simulink model "CPGGait2"  (R2021a)
settings: Solver=FixedStepDiscrete  StartTime=0.0  StopTime=30  FixedStep=deltaT  RelTol=1e-3  EnableMultiTasking=on
InitFcn:
  | deltaT = 0.02; % this model runs at 50 Hz
  | 
  | DEVICENAME  = 'COM4'; % COM port that USB2Dynamixel is plugged into
  | % NOTE: go to Device Manager to make sure device name is correct
  | 
  | lib_name = ''; % initialize library name
  | % get library name based on computer:
  | if strcmp(computer, 'PCWIN')
  |   lib_name = 'dxl_x86_c';
  | elseif strcmp(computer, 'PCWIN64')
  |   lib_name = 'dxl_x64_c';
  | elseif strcmp(computer, 'GLNX86')
  |   lib_name = 'libdxl_x86_c';
  | elseif strcmp(computer, 'GLNXA64')
  |   lib_name = 'libdxl_x64_c';
  | elseif strcmp(computer, 'MACI64')
  |   lib_name = 'libdxl_mac_c';
  | end
  | 
  | % Load Libraries
  | if ~libisloaded(lib_name)
  |     [notfound, warnings] = loadlibrary(lib_name, 'dynamixel_sdk.h', 'addheader', 'port_handler.h', 'addheader', 'packet_handler.h', 'addheader','group_sync_write.h');
  | end
  | 
  | % Control table address
  | ADDR_MX_TORQUE_ENABLE       = 24;           % Control table address is different in Dynamixel model
  | ADDR_MX_GOAL_POSITION       = 30;
  | ADDR_MX_PRESENT_POSITION    = 36;
  | 
  | % Data Byte Length
  | LEN_MX_GOAL_POSITION        = 2;
  | 
  | % Protocol version
  | PROTOCOL_VERSION            = 1.0;          % See which protocol version is used in the Dynamixel
  | 
  | % Default setting
  | BAUDRATE                    = 1000000;
  | 
  | TORQUE_ENABLE               = 1;            % Value for enabling the torque
  | TORQUE_DISABLE              = 0;            % Value for disabling the torque
  | DXL_MINIMUM_POSITION_VALUE  = 100;          % Dynamixel will rotate between this value
  | DXL_MAXIMUM_POSITION_VALUE  = 500;         % and this value (note that the Dynamixel would not move when the position value is out of movable range. Check e-manual about the range of the Dynamixel you use.)
  | DXL_MOVING_STATUS_THRESHOLD = 10;           % Dynamixel moving status threshold
  | 
  | COMM_SUCCESS                = 0;            % Communication Success result value
  | COMM_TX_FAIL                = -1001;        % Communication Tx Failed
  | 
  | % Initialize PortHandler Structs
  | % Set the port path
  | % Get methods and members of PortHandlerLinux or PortHandlerWindows
  | port_num = portHandler(DEVICENAME);
  | 
  | % Initialize PacketHandler Structs
  | packetHandler();
  | 
  | dxl_comm_result = COMM_TX_FAIL;             % Communication result
  | 
  | dxl_error = 0;                              % Dynamixel error
  | dxl_present_position = 0;                   % Present position
  | 
  | % Initialize Groupsyncwrite instance
  | group_num = groupSyncWrite(port_num, PROTOCOL_VERSION, ADDR_MX_GOAL_POSITION, LEN_MX_GOAL_POSITION);
  | 
  | % Open port
  | if (openPort(port_num))
  |     fprintf('Succeeded to open the port!\n');
  | else
  |     unloadlibrary(lib_name);
  |     fprintf('Failed to open the port!\n');
  |     input('Press any key to terminate...\n');
  |     dxl_error = 1000;
  |     return;
  | end
  | 
  | % Set port baudrate
  | if (setBaudRate(port_num, BAUDRATE))
  |     fprintf('Succeeded to change the baudrate!\n');
  | else
  |     unloadlibrary(lib_name);
  |     fprintf('Failed to change the baudrate!\n');
  |     input('Press any key to terminate...\n');
  |     dxl_error = 2000;
  |     return;
  | end
  | 
  | % set ID numbers of the the Dynamixels to be controlled:
  | % (even numbers are left side of body, odd numbers are right side)
  | ID01                     = 1;            % Dynamixel IDs for sagittal shoulders
  | ID02                     = 2;
  | ID03                     = 3;            % Dynamixel IDs for frontal shoulders
  | ID04                     = 4;
  | ID05                     = 5;            % Dynamixel IDs for elbows
  | ID06                     = 6;
  | ID07                     = 7;            % Dynamixel IDs for transverse hips
  | ID08                     = 8;
  | ID09                     = 9;            % Dynamixel IDs for frontal hips
  | ID10                     = 10;
  | ID11                     = 11;            % Dynamixel IDs for sagittal hips
  | ID12                     = 12;
  | ID13                     = 13;            % Dynamixel IDs for knees
  | ID14                     = 14;
  | ID15                     = 15;            % Dynamixel IDs for sagittal ankles
  | ID16                     = 16;
  | ID17                     = 17;            % Dynamixel IDs for frontal ankles
  | ID18                     = 18;
  | 
  | %% Enable Dynamixel Torques and connect Dynamixels
  | write1ByteTxRx(port_num, PROTOCOL_VERSION, ID01, ADDR_MX_TORQUE_ENABLE, TORQUE_ENABLE);
  | write1ByteTxRx(port_num, PROTOCOL_VERSION, ID02, ADDR_MX_TORQUE_ENABLE, TORQUE_ENABLE);
  | write1ByteTxRx(port_num, PROTOCOL_VERSION, ID03, ADDR_MX_TORQUE_ENABLE, TORQUE_ENABLE);
  | write1ByteTxRx(port_num, PROTOCOL_VERSION, ID04, ADDR_MX_TORQUE_ENABLE, TORQUE_ENABLE);
  | write1ByteTxRx(port_num, PROTOCOL_VERSION, ID05, ADDR_MX_TORQUE_ENABLE, TORQUE_ENABLE);
  | write1ByteTxRx(port_num, PROTOCOL_VERSION, ID06, ADDR_MX_TORQUE_ENABLE, TORQUE_ENABLE);
  | write1ByteTxRx(port_num, PROTOCOL_VERSION, ID07, ADDR_MX_TORQUE_ENABLE, TORQUE_ENABLE);
  | write1ByteTxRx(port_num, PROTOCOL_VERSION, ID08, ADDR_MX_TORQUE_ENABLE, TORQUE_ENABLE);
  | write1ByteTxRx(port_num, PROTOCOL_VERSION, ID09, ADDR_MX_TORQUE_ENABLE, TORQUE_ENABLE);
  | write1ByteTxRx(port_num, PROTOCOL_VERSION, ID10, ADDR_MX_TORQUE_ENABLE, TORQUE_ENABLE);
  | write1ByteTxRx(port_num, PROTOCOL_VERSION, ID11, ADDR_MX_TORQUE_ENABLE, TORQUE_ENABLE);
  | write1ByteTxRx(port_num, PROTOCOL_VERSION, ID12, ADDR_MX_TORQUE_ENABLE, TORQUE_ENABLE);
  | write1ByteTxRx(port_num, PROTOCOL_VERSION, ID13, ADDR_MX_TORQUE_ENABLE, TORQUE_ENABLE);
  | write1ByteTxRx(port_num, PROTOCOL_VERSION, ID14, ADDR_MX_TORQUE_ENABLE, TORQUE_ENABLE);
  | write1ByteTxRx(port_num, PROTOCOL_VERSION, ID15, ADDR_MX_TORQUE_ENABLE, TORQUE_ENABLE);
  | write1ByteTxRx(port_num, PROTOCOL_VERSION, ID16, ADDR_MX_TORQUE_ENABLE, TORQUE_ENABLE);
  | write1ByteTxRx(port_num, PROTOCOL_VERSION, ID17, ADDR_MX_TORQUE_ENABLE, TORQUE_ENABLE);
  | write1ByteTxRx(port_num, PROTOCOL_VERSION, ID18, ADDR_MX_TORQUE_ENABLE, TORQUE_ENABLE);
  | dxl_comm_result = getLastTxRxResult(port_num, PROTOCOL_VERSION);
  | dxl_error = getLastRxPacketError(port_num, PROTOCOL_VERSION);
  | if dxl_comm_result ~= COMM_SUCCESS
  |     fprintf('%s\n', getTxRxResult(PROTOCOL_VERSION, dxl_comm_result));
  | elseif dxl_error ~= 0
  |     fprintf('%s\n', getRxPacketError(PROTOCOL_VERSION, dxl_error));
  | else
  |     fprintf('Dynamixel has been successfully connected \n');
  | end
  | 
  | % the variable 'qinitial' is an 18x1 vector of initial joint angles for the
  | % robot (in DEGREES!); adjust for your robot!
  | if exist('qinitial','var') ~= 1
  | qinitial = (180/pi)*[0.2;1.19321189006954;-1.72642378013908;0.413211890069541;0.15;0;0;-0.15;0.413211890069541;-1.72642378013908;1.19321189006954;0.20;0.1683;0.349;-0.051;0.1683;-0.349;0.997];
  | end
StopFcn:
  | %% Disable Dynamixel Torque and close program
  | write1ByteTxRx(port_num, PROTOCOL_VERSION, ID01, ADDR_MX_TORQUE_ENABLE, TORQUE_DISABLE);
  | write1ByteTxRx(port_num, PROTOCOL_VERSION, ID02, ADDR_MX_TORQUE_ENABLE, TORQUE_DISABLE);
  | write1ByteTxRx(port_num, PROTOCOL_VERSION, ID03, ADDR_MX_TORQUE_ENABLE, TORQUE_DISABLE);
  | write1ByteTxRx(port_num, PROTOCOL_VERSION, ID04, ADDR_MX_TORQUE_ENABLE, TORQUE_DISABLE);
  | write1ByteTxRx(port_num, PROTOCOL_VERSION, ID05, ADDR_MX_TORQUE_ENABLE, TORQUE_DISABLE);
  | write1ByteTxRx(port_num, PROTOCOL_VERSION, ID06, ADDR_MX_TORQUE_ENABLE, TORQUE_DISABLE);
  | write1ByteTxRx(port_num, PROTOCOL_VERSION, ID07, ADDR_MX_TORQUE_ENABLE, TORQUE_DISABLE);
  | write1ByteTxRx(port_num, PROTOCOL_VERSION, ID08, ADDR_MX_TORQUE_ENABLE, TORQUE_DISABLE);
  | write1ByteTxRx(port_num, PROTOCOL_VERSION, ID09, ADDR_MX_TORQUE_ENABLE, TORQUE_DISABLE);
  | write1ByteTxRx(port_num, PROTOCOL_VERSION, ID10, ADDR_MX_TORQUE_ENABLE, TORQUE_DISABLE);
  | write1ByteTxRx(port_num, PROTOCOL_VERSION, ID11, ADDR_MX_TORQUE_ENABLE, TORQUE_DISABLE);
  | write1ByteTxRx(port_num, PROTOCOL_VERSION, ID12, ADDR_MX_TORQUE_ENABLE, TORQUE_DISABLE);
  | write1ByteTxRx(port_num, PROTOCOL_VERSION, ID13, ADDR_MX_TORQUE_ENABLE, TORQUE_DISABLE);
  | write1ByteTxRx(port_num, PROTOCOL_VERSION, ID14, ADDR_MX_TORQUE_ENABLE, TORQUE_DISABLE);
  | write1ByteTxRx(port_num, PROTOCOL_VERSION, ID15, ADDR_MX_TORQUE_ENABLE, TORQUE_DISABLE);
  | write1ByteTxRx(port_num, PROTOCOL_VERSION, ID16, ADDR_MX_TORQUE_ENABLE, TORQUE_DISABLE);
  | write1ByteTxRx(port_num, PROTOCOL_VERSION, ID17, ADDR_MX_TORQUE_ENABLE, TORQUE_DISABLE);
  | write1ByteTxRx(port_num, PROTOCOL_VERSION, ID18, ADDR_MX_TORQUE_ENABLE, TORQUE_DISABLE);
  | dxl_comm_result = getLastTxRxResult(port_num, PROTOCOL_VERSION);
  | dxl_error = getLastRxPacketError(port_num, PROTOCOL_VERSION);
  |    if dxl_comm_result ~= COMM_SUCCESS
  |        fprintf('%s\n', getTxRxResult(PROTOCOL_VERSION, dxl_comm_result));
  |    elseif dxl_error ~= 0
  |        fprintf('%s\n', getRxPacketError(PROTOCOL_VERSION, dxl_error));
  |    end
  | 
  | % Close port
  | closePort(port_num);
  | 
  | % Unload Library
  | unloadlibrary(lib_name);
  | 
  | q = q'; qdes = qdes';
undefined symbols (not defined in the file or in its folder): k
libraries: realtime_pacer_lib x1
PauseFcn:
  | %IMUscript;
  | xx = timer('ExecutionMode','singleShot','StartDelay',0.001,'TimerFcn','set_param(bdroot, "SimulationCommand","continue")'); start(xx)
settings Model: SimulationMode=external  SILPILModeSetting=veronly  ExtModeTrigDuration=2  Creator=The MathWorks, Inc.  LastModifiedBy=JerryLee
settings SolverCC: AlgebraicLoopSolver=TrustRegion  PositivePriorityOrder=on
settings DataIOCC: SaveFormat=Array  ReturnWorkspaceOutputs=off
settings OptimizationCC: ExpressionDepthLimit=2147483647  LifeSpan=Inf  MaxStackSize=64
settings DebuggingCC: UnderspecifiedInitializationDetection=Classic  MergeDetectMultiDrivingBlocksExec=none  FcnCallInpInsideContextMsg=warning  AllowSymbolicDim=off  StateNameClashWarn=warning  SFUnexpectedBacktrackingDiag=warning  SFNoUnconditionalDefaultTransitionDiag=warning  SFExecutionAtInitializationDiag=none  SFMachineParentedDataDiag=warning  UnderSpecifiedDimensionMsg=warning  ArithmeticOperatorsInVariantConditions=warning
settings HardwareCC: ProdBitPerInt=16  ProdBitPerPointer=16  ProdBitPerSizeT=16  ProdBitPerPtrDiffT=16  ProdLargestAtomicFloat=None  ProdWordSize=8  ProdHWDeviceType=Atmel->AVR
settings ModelReferenceCC: PropagateSignalLabelsOutOfModel=off
settings SFSimCC: SimUseLocalCustomCode=off  MATLABDynamicMemAlloc=off  CustomCodeUndefinedFunction=UseInterfaceOnly
settings RTWCC: SystemTargetFile=ert.tlc  HardwareBoard=Arduino Nano 3.0  TemplateMakefile=ert_default_tmf  GenerateReport=on  RTWVerbose=off  RTWUseLocalCustomCode=off  Toolchain=Arduino AVR  BuildConfiguration=Faster Runs  LaunchReport=on
settings CodeAppCC: ForceParamTrailComments=on  OperatorAnnotations=on  MangleLength=10  StateflowObjectComments=on  MATLABSourceComments=on
settings ERTTargetCC: MultiwordLength=2048  ERTCustomFileBanners=off  SupportContinuousTime=on  SupportNonInlinedSFcns=on  RemoveResetFunc=off  SupportVariableSizeSignals=on  ModelStepFunctionPrototypeControlCompliant=off  ExtModeStaticAllocSize=250
settings ConfigComp: CovMetricSettings=dw  CovSaveCumulativeToWorkspaceVar=on  CovSaveSingleToWorkspaceVar=on  CovExternalEMLEnable=off

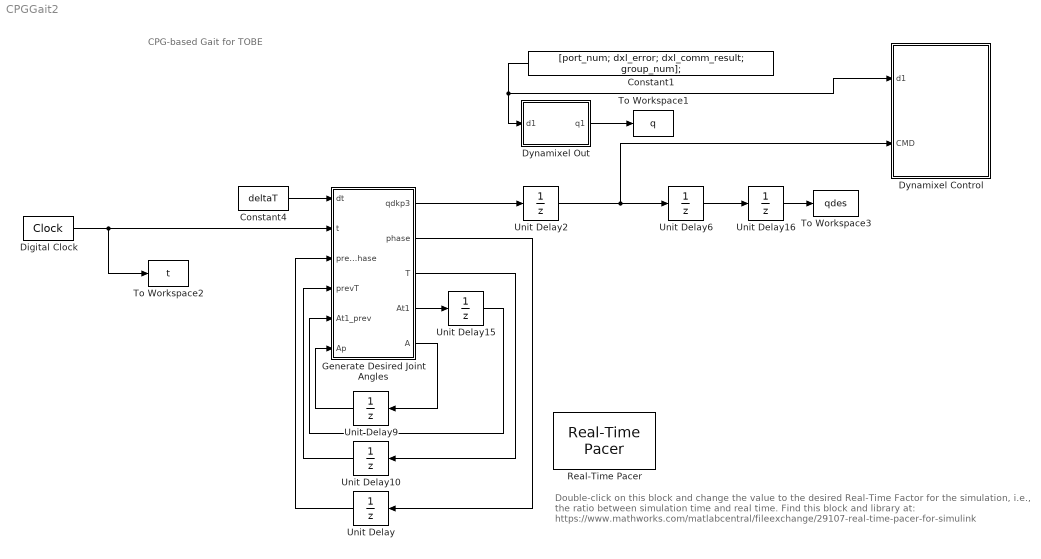
== system CPGGait2 ==
  note: CPG-based Gait for TOBE
  note: Double-click on this block and change the value to the desired Real-Time Factor for the simulation,
      | i.e., the ratio between simulation time and real time.
      |
      | Find this block and library at:
      | https://www.mathworks.com/matlabcentral/fileexchange/29107-real-time-pacer-for-simulink
  Constant1 : Constant  Value=[port_num; dxl_error; dxl_comm_result; group_num];
  Constant4 : Constant  Value=deltaT
  Digital Clock : DigitalClock  SampleTime=deltaT
  Dynamixel Control : MATLAB Function  TreatAsAtomicUnit=on
  Dynamixel Out : MATLAB Function  TreatAsAtomicUnit=on
  Generate Desired Joint Angles : MATLAB Function  TreatAsAtomicUnit=on
  Real-Time Pacer : realtime_pacer_lib/Real-Time Pacer  simTimePerRealTime=1
  To Workspace1 : ToWorkspace  VariableName=q  SampleTime=deltaT
  To Workspace2 : ToWorkspace  VariableName=t  SampleTime=-1
  To Workspace3 : ToWorkspace  VariableName=qdes  SampleTime=deltaT
  Unit Delay : UnitDelay  InitialCondition=0.6+0.2666*pi  SampleTime=deltaT  HasFrameUpgradeWarning=on
  Unit Delay10 : UnitDelay  InitialCondition=2.2  SampleTime=deltaT  HasFrameUpgradeWarning=on
  Unit Delay15 : UnitDelay  SampleTime=deltaT*k  HasFrameUpgradeWarning=on
  Unit Delay16 : UnitDelay  InitialCondition=qinitial  SampleTime=deltaT  HasFrameUpgradeWarning=on
  Unit Delay2 : UnitDelay  InitialCondition=qinitial  SampleTime=deltaT  HasFrameUpgradeWarning=on
  Unit Delay6 : UnitDelay  InitialCondition=qinitial  SampleTime=deltaT  HasFrameUpgradeWarning=on
  Unit Delay9 : UnitDelay  InitialCondition=[0;-0.24;0]  SampleTime=deltaT  HasFrameUpgradeWarning=on
  wires:
  Generate Desired Joint Angles/2(phase) -> Unit Delay/1
  Unit Delay/1 -> Generate Desired Joint Angles/3(prevphase)
  Unit Delay2/1 -> Unit Delay6/1, Dynamixel Control/2(CMD)
  Constant4/1 -> Generate Desired Joint Angles/1(dt)
  Digital Clock/1 -> Generate Desired Joint Angles/2(t), To Workspace2/1
  Dynamixel Out/1(q1) -> To Workspace1/1
  Constant1/1 -> Dynamixel Out/1(d1), Dynamixel Control/1(d1)
  Generate Desired Joint Angles/5(A) -> Unit Delay9/1
  Unit Delay9/1 -> Generate Desired Joint Angles/6(Ap)
  Generate Desired Joint Angles/3(T) -> Unit Delay10/1
  Unit Delay10/1 -> Generate Desired Joint Angles/4(prevT)
  Generate Desired Joint Angles/4(At1) -> Unit Delay15/1
  Unit Delay15/1 -> Generate Desired Joint Angles/5(At1_prev)
  Unit Delay6/1 -> Unit Delay16/1
  Generate Desired Joint Angles/1(qdkp3) -> Unit Delay2/1
  Unit Delay16/1 -> To Workspace3/1

== matlab function CPGGait2/Generate Desired Joint Angles ==
  data: qdkp3 output; dt input; t input; prevphase input; phase output size=1; prevT input; At1_prev input; T output size=1; At1 output; Ap input; A output
function [qdkp3,phase,T,At1,A] = getjoints(dt,t,prevphase,prevT,At1_prev,Ap)
%#codegen
% based on Missura PhD thesis, 2015 and 
% Capture Steps paper by Missura, Bennewitz, Behnke, 2020

tstart = 2; % robot stays at 'qinitial' pose until 'tstart'
tstop = 27.3; % robot stops gait sequence, moves to 'qinitial' pose at tstop
Tinit = 2; % initial step time

% step size
Sx = -0.8; % since kx = 0.5, the absolute value of this should probably not exceed 2
S = [Sx;0;0]; % setting the other parameters to zero limits stepping to forward/backward direction only

% configuration parameters:
K20 = 3.5;
K21 = 0.2;
K22 = 0.2;
K23 = 0.2;
K25 = 3;
Sy_min = 0.05;
Sy_max = 0.3;
kx = 0.3;
kphi = 0.2;

%% Compute command positions for joints
T = prevT - dt; % decrement time to swing foot touchdown
if T <= 0 % if this value reaches zero (the foot should be touching down)
    T = Tinit; % reset time for new swing foot to touch down
end

% compute step frequency 'omega' based on 'prevphase' and T 
if prevphase > 0
    nu = pi - prevphase;
else
    nu = -prevphase;
end
omega = nu/(pi*T);

% 'omega' should be bounded, since it can get large when T approaches zero
if omega > K25
    omega = K25; 
end

% update phase ('phase' progresses from -pi to pi, then resets back to -pi)
phase = prevphase + omega*pi*dt; 

% reset 'phase' to -pi, if necessary 
if phase >= pi
    phase = -pi;
end

% transform desired step size S to step size in trunk frame 'St'
R = [cos(-0.5*S(3)),-sin(-0.5*S(3));sin(-0.5*S(3)),cos(-0.5*S(3))];
SxSy = R*S(1:2);
St = [SxSy;S(3)];

% find swing amplitude target 'At'
if -sign(phase)*St(2) > Sy_min
    At1 = -sign(phase)*(abs(St(2))-Sy_min)/(Sy_max-Sy_min);
else
    At1 = At1_prev;
end
At = [At1;kx*St(1);kphi*St(3)];

% if time has elapsed past 'tstop'...
if t >= tstop
    At = [0;0;0]; % stop walking from current position
end

% if the target swing amplitude is too large, set it to a lower value 
if norm(At,K20) > 1
    At = At/norm(At,K20);
end

% move swing amplitude closer to target swing amplitude by bounded increments
dA1 = min(max(At(1)-Ap(1),-K21*dt),K21*dt);
dA2 = min(max(At(2)-Ap(2),-K22*dt),K22*dt);
dA3 = min(max(At(3)-Ap(3),-K23*dt),K23*dt);

A = At + 0*(Ap + [dA1;dA2;dA3]); % update swing amplitude 
% (here, I am using A = At. To use the algorithm as originally designed,
% delete 'At' and the zero multiplier from this equation.)

% compute desired joint angles
[eta,phi_leg,phi_foot] = LegMotion(A,phase);
angles = LegInterface(eta,phi_leg,phi_foot);

% set phase to initial value 
if t > tstop || t < tstart
    phase = 0.6 - 1.05*pi;
    A = [0;-0.24;0];
    angles = [0.2;1.19321189006954;-1.72642378013908;0.413211890069541;0.15;0;0;-0.15;0.413211890069541;-1.72642378013908;1.19321189006954;0.2];
end

% assign desired joint trajectories for arms
sag = -pi/8; elb = pi/6; 
phase1 = phase - 0.6; % this offsets the arm motions to better align them with the leg motions 
Lsag = sag*sin(phase1);
Rsag = sag*sin(phase1);
Lelb = elb*cos(phase1+pi) - elb;
Relb = elb*cos(phase1+pi) + elb;
Lfro = pi/9; Rfro = -pi/9;
arms = [Lsag;Lfro;Lelb;Rsag;Rfro;Relb];

% Set command positions for joints
qdkp3 = (180/pi)*[angles;arms];

== matlab function CPGGait2/Dynamixel Control ==
  data: d1 input; CMD input
function runmotors(d1,CMD)
%#codegen

% this MEX file is based on the RunMotors.m file
coder.extrinsic('RunMotors_mex');

port_num = d1(1);
group_num = d1(4);

% convert joint angle command to 10-bit servo command
qcmd = servoangles((pi/180)*CMD);

RunMotors_mex(port_num,group_num,qcmd);

== matlab function CPGGait2/Dynamixel Out ==
  data: d1 input; q1 output
function q1 = readmotors(d1)
%#codegen

% this block reads the Dynamixel motor positions:

% the MEX file used here is based on the ReadMotors.m file
coder.extrinsic('ReadMotors_mex');

port_num = d1(1);

q1 = zeros(18,1); % initialize the joint angle vector size
q1 = ReadMotors_mex(port_num);
